simulink model "open_loop_state_estimation"  (R2018b)
settings: Solver=ode2  StartTime=0.0  StopTime=100  FixedStep=0.002  RelTol=1e-3  EnableMultiTasking=on
model workspace (MAT data in the model file):
  m = 1000
undefined symbols (not defined in the file): activate_VariableFriction, sigbuilder_block, tpa_map_Reference, tS, x0_vehiclepose_stm
libraries: simulink x6
settings Model: DataDictionary=controller_dev.sldd  PauseTimes=9.280  Creator=wischnewski  LastModifiedBy=ga25xiw
settings SolverCC: AutoInsertRateTranBlk=on
settings DataIOCC: SaveFormat=StructureWithTime
settings OptimizationCC: BlockReduction=off  DefaultParameterBehavior=Inlined  EnhancedBackFolding=on  PassReuseOutputArgsAs=Individual arguments  OptimizeBlockOrder=speed  DifferentSizesBufferReuse=on  OptimizationCustomize=off
settings DebuggingCC: ParameterTunabilityLossMsg=error
settings HardwareCC: ProdBitPerPointer=32  ProdBitPerSizeT=32  ProdBitPerPtrDiffT=32  ProdLargestAtomicFloat=None  ProdWordSize=32  ProdLongLongMode=on  ProdHWDeviceType=Generic->32-bit x86 compatible
settings ModelReferenceCC: ModelReferenceMinAlgLoopOccurrences=on
settings SFSimCC: SimUseLocalCustomCode=off  MATLABDynamicMemAlloc=off
settings RTWCC: SystemTargetFile=ert.tlc  TemplateMakefile=ert_default_tmf  GenerateReport=on  RTWUseLocalCustomCode=off  IncludeHyperlinkInReport=on  LaunchReport=on  TargetLang=C++  GenerateTraceInfo=on  GenerateTraceReport=on  GenerateTraceReportSl=on  GenerateTraceReportSf=on  GenerateTraceReportEml=on
settings CodeAppCC: ForceParamTrailComments=on  IgnoreCustomStorageClasses=off  OperatorAnnotations=on  SimulinkDataObjDesc=on  SFDataObjDesc=on  InsertBlockDesc=on
settings ERTTargetCC: TargetLangStandard=C++03 (ISO)  GenerateSampleERTMain=on  MultiInstanceERTCode=on  CodeInterfacePackaging=C++ class  InlinedParameterPlacement=NonHierarchical  RootIOFormat=Structure reference  ERTCustomFileTemplate=example_file_process.tlc

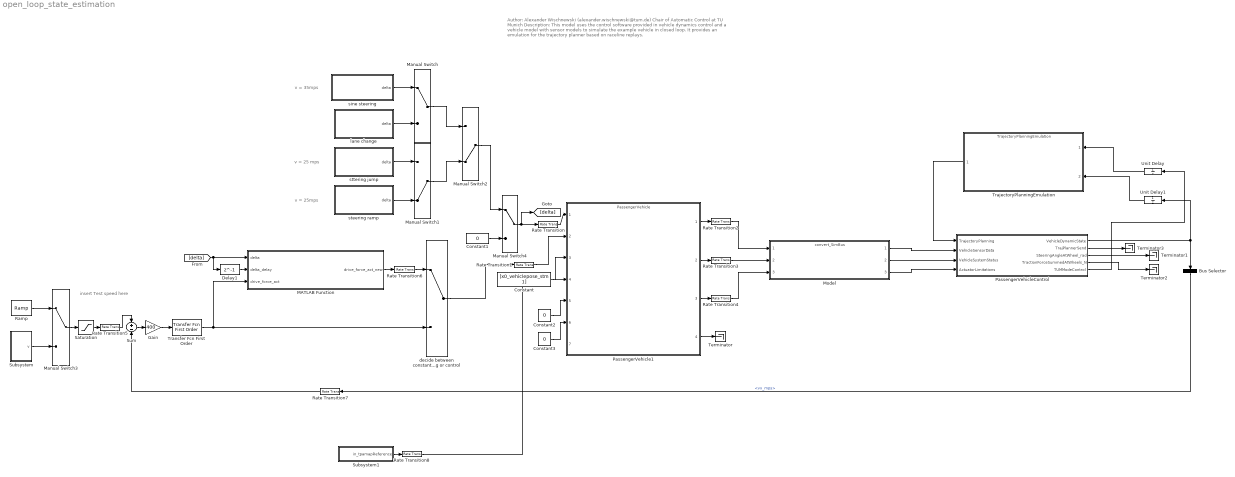
== system open_loop_state_estimation ==
  note: v = 25mps
  note: v = 35mps
  note: v = 25 mps
  note: insert Test speed here
  note: Author: Alexander Wischnewski (alexander.wischnewski@tum.de)
      | Chair of Automatic Control at TU Munich
      |
      | Description: This model uses the control software provided in vehicle dynamics control and a vehicle model
      | with sensor models to simulate the example vehicle in closed loop. It provides an emulation for the trajectory planner based on raceline replays.
  Bus Selector : BusSelector  OutputSignals=vx_mps
  Constant : Constant  Value=[x0_vehiclepose_stm 1]
  Constant1 : Constant  Value=0
  Constant2 : Constant  Value=0
  Constant3 : Constant  Value=0
  Delay1 : Delay  DelayLength=1
  Gain : Gain  Gain=400
  MATLAB Function : MATLAB Function  TreatAsAtomicUnit=on
  Manual Switch : ManualSwitch
  Manual Switch1 : ManualSwitch  CurrentSetting=0
  Manual Switch2 : ManualSwitch  CurrentSetting=0
  Manual Switch3 : ManualSwitch
  Manual Switch4 : ManualSwitch
  Model : ModelReference  ModelNameDialog=convert_SimBus.slx  SimulationMode=Normal  ModelReferenceVersion=1.818
  PassengerVehicle1 : ModelReference  ModelNameDialog=PassengerVehicle  SimulationMode=Normal  ModelReferenceVersion=1.933
  PassengerVehicleControl : Subsystem
  Ramp : simulink/Sources/Ramp  slope=8  start=0  InitialOutput=0.1
  Rate Transition{,1..8} (9 alike) : RateTransition
  Saturation : Saturate  UpperLimit=25  LowerLimit=0
  Subsystem : Subsystem
  Subsystem1 : Subsystem
  Sum : Sum  Inputs=+-
  Terminator{,1..3} (4 alike) : Terminator
  TrajectoryPlanningEmulation : ModelReference  ModelNameDialog=TrajectoryPlanningEmulation.slx  SimulationMode=Normal  ModelReferenceVersion=1.855
  Transfer Fcn First Order : simulink/Discrete/Transfer Fcn First Order  PoleZ=exp(-tS/1)  ICPrevOutput=0.0  DoSatur=off
      settings: SourceProductName=Simulink
  Unit Delay : UnitDelay  SampleTime=-1
  Unit Delay1 : UnitDelay  SampleTime=-1
  "decide between constant torque while steering or control " : ManualSwitch
  lane change : Subsystem
  sine steering : Subsystem
  steering ramp : Subsystem
  sttering jump : Subsystem
  wires:
  TrajectoryPlanningEmulation/1 -> PassengerVehicleControl/1(TrajectoryPlanning)
  PassengerVehicleControl/1(VehicleDynamicState) -> Unit Delay1/1, Bus Selector/1
  Unit Delay/1 -> TrajectoryPlanningEmulation/1
  Unit Delay1/1 -> TrajectoryPlanningEmulation/2
  PassengerVehicle1/3 -> Rate Transition4/1
  PassengerVehicle1/2 -> Rate Transition3/1
  PassengerVehicle1/1 -> Rate Transition2/1
  Constant/1 -> PassengerVehicle1/3
  Rate Transition/1 -> PassengerVehicle1/1
  Rate Transition1/1 -> PassengerVehicle1/2
  PassengerVehicleControl/3(SteeringAngleAtWheel_rad) -> Terminator1/1
  Sum/1 -> Gain/1
  PassengerVehicleControl/4(TractionForceSummedAtWheels_N) -> Terminator2/1
  Bus Selector/1 -> Rate Transition7/1  "<vx_mps>"
  Gain/1 -> Transfer Fcn First Order/1
  Saturation/1 -> Rate Transition5/1
  Rate Transition5/1 -> Sum/1
  sine steering/1(delta) -> Manual Switch/1
  lane change/1(delta) -> Manual Switch/2
  sttering jump/1(delta) -> Manual Switch1/1
  steering ramp/1(delta) -> Manual Switch1/2
  Manual Switch1/1 -> Manual Switch2/2
  Manual Switch/1 -> Manual Switch2/1
  Manual Switch3/1 -> Saturation/1
  Ramp/1 -> Manual Switch3/1
  Manual Switch4/1 -> [delta], Rate Transition/1
  Manual Switch2/1 -> Manual Switch4/1
  Constant1/1 -> Manual Switch4/2
  Subsystem/1("v ") -> Manual Switch3/2
  "decide between constant torque while steering or control "/1 -> Rate Transition1/1
  Transfer Fcn First Order/1 -> "decide between constant torque while steering or control "/2, MATLAB Function/3(drive_force_act)
  [delta] -> MATLAB Function/1(delta), Delay1/1
  Delay1/1 -> MATLAB Function/2(delta_delay)
  MATLAB Function/1(drive_force_act_new) -> Rate Transition6/1
  Rate Transition6/1 -> "decide between constant torque while steering or control "/1
  Rate Transition7/1 -> Sum/2
  PassengerVehicle1/4 -> Terminator/1
  Subsystem1/1(in_tpamapReference) -> Rate Transition8/1
  Rate Transition8/1 -> PassengerVehicle1/4
  Rate Transition2/1 -> Model/1
  Model/1 -> PassengerVehicleControl/2(VehicleSensorData)
  Rate Transition3/1 -> Model/2
  Rate Transition4/1 -> Model/3
  Model/2 -> PassengerVehicleControl/3(VehicleSystemStatus)
  Model/3 -> PassengerVehicleControl/4(ActuatorLimitations)
  Constant2/1 -> PassengerVehicle1/5
  Constant3/1 -> PassengerVehicle1/6
  PassengerVehicleControl/5(TUMModeControl) -> Unit Delay/1
  PassengerVehicleControl/2(TrajPlannerSend) -> Terminator3/1

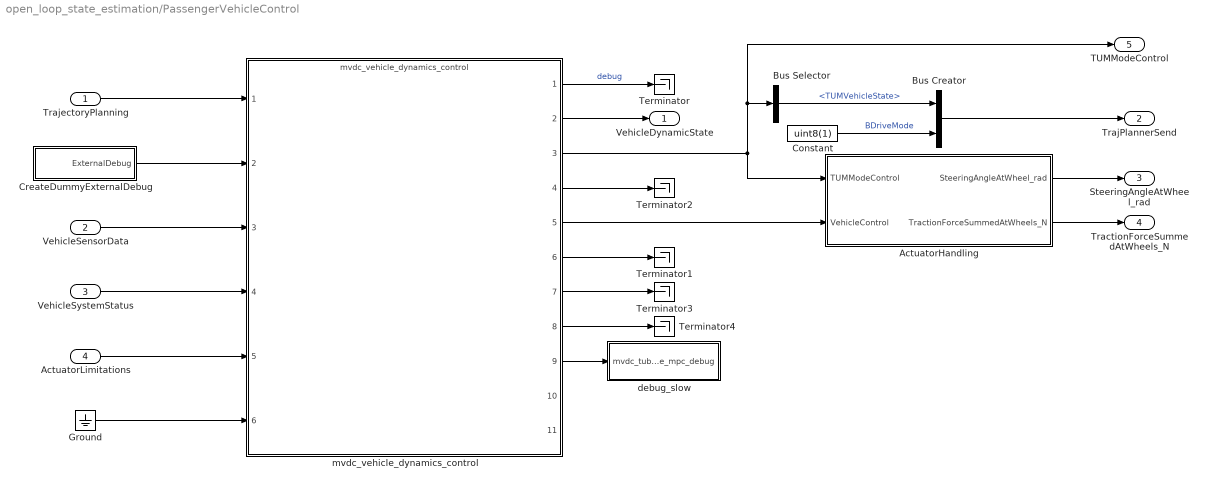
== system open_loop_state_estimation/PassengerVehicleControl ==
  TrajectoryPlanning : Inport
  VehicleSensorData : Inport  Port=2
  VehicleSystemStatus : Inport  Port=3
  ActuatorLimitations : Inport  Port=4
  ActuatorHandling : Subsystem
  Bus Creator : BusCreator  Inputs=2
  Bus Selector : BusSelector  OutputSignals=TUMVehicleState
  Constant : Constant  Value=uint8(1)
  CreateDummyExternalDebug : Subsystem
  Ground : Ground
  Terminator{,1..4} (5 alike) : Terminator
  debug_slow : Subsystem
  mvdc_vehicle_dynamics_control : ModelReference  ModelNameDialog=mvdc_vehicle_dynamics_control  SimulationMode=Normal  ModelReferenceVersion=1.789
  VehicleDynamicState : Outport
  TrajPlannerSend : Outport  Port=2
  SteeringAngleAtWheel_rad : Outport  Port=3
  TractionForceSummedAtWheels_N : Outport  Port=4
  TUMModeControl : Outport  Port=5  OutDataTypeStr=Bus: TUMModeControl
  wires:
  mvdc_vehicle_dynamics_control/1 -> Terminator/1  "debug"
  VehicleSystemStatus/1 -> mvdc_vehicle_dynamics_control/4
  ActuatorLimitations/1 -> mvdc_vehicle_dynamics_control/5
  VehicleSensorData/1 -> mvdc_vehicle_dynamics_control/3
  TrajectoryPlanning/1 -> mvdc_vehicle_dynamics_control/1
  mvdc_vehicle_dynamics_control/5 -> ActuatorHandling/2(VehicleControl)
  mvdc_vehicle_dynamics_control/6 -> Terminator1/1
  ActuatorHandling/2(TractionForceSummedAtWheels_N) -> TractionForceSummedAtWheels_N/1
  ActuatorHandling/1(SteeringAngleAtWheel_rad) -> SteeringAngleAtWheel_rad/1
  mvdc_vehicle_dynamics_control/7 -> Terminator3/1
  mvdc_vehicle_dynamics_control/8 -> Terminator4/1
  Bus Selector/1 -> Bus Creator/1  "<TUMVehicleState>"
  Constant/1 -> Bus Creator/2  "BDriveMode"
  Bus Creator/1 -> TrajPlannerSend/1
  mvdc_vehicle_dynamics_control/2 -> VehicleDynamicState/1
  mvdc_vehicle_dynamics_control/9 -> debug_slow/1(mvdc_tube_mpc_debug)
  mvdc_vehicle_dynamics_control/3 -> ActuatorHandling/1(TUMModeControl), TUMModeControl/1, Bus Selector/1
  mvdc_vehicle_dynamics_control/4 -> Terminator2/1
  CreateDummyExternalDebug/1(ExternalDebug) -> mvdc_vehicle_dynamics_control/2
  Ground/1 -> mvdc_vehicle_dynamics_control/6

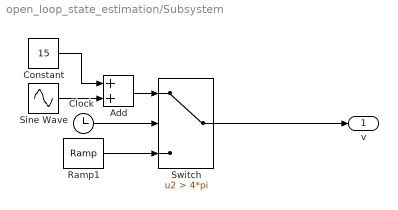
== system open_loop_state_estimation/Subsystem ==
  Add : Sum
  Clock : Clock
  Constant : Constant  Value=15
  Ramp1 : simulink/Sources/Ramp  slope=8  start=0  InitialOutput=0.1
  Sine Wave : Sin  Amplitude=25  SampleTime=0
  Switch : Switch  Criteria=u2 > Threshold  Threshold=4*pi
  "v " : Outport
  wires:
  Clock/1 -> Switch/2
  Switch/1 -> "v "/1
  Ramp1/1 -> Switch/3
  Add/1 -> Switch/1
  Sine Wave/1 -> Add/2
  Constant/1 -> Add/1

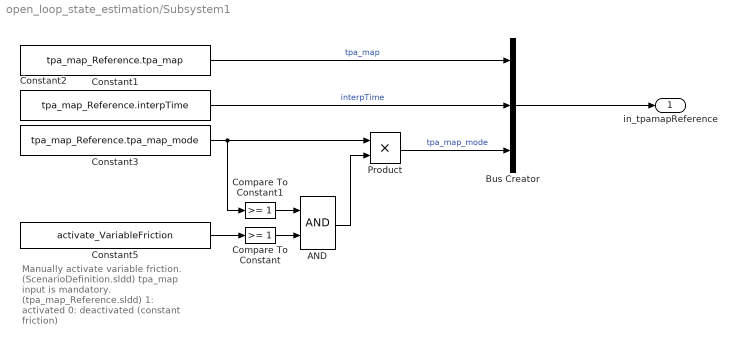
== system open_loop_state_estimation/Subsystem1 ==
  note: Manually activate variable friction.
      | (ScenarioDefinition.sldd)      tpa_map input is mandatory. (tpa_map_Reference.sldd)
      |
      | 1: activated
      | 0: deactivated (constant friction)
  AND : Logic  AllPortsSameDT=off  OutDataTypeStr=boolean
  Bus Creator : BusCreator  Inputs=3  OutDataTypeStr=Bus: tpamapReference
  Compare To Constant : simulink/Logic and Bit Operations/Compare To Constant  relop=>=  const=1  OutDataTypeStr=boolean
  Compare To Constant1 : simulink/Logic and Bit Operations/Compare To Constant  relop=>=  const=1  OutDataTypeStr=boolean
  Constant1 : Constant  Value=tpa_map_Reference.tpa_map
  Constant2 : Constant  Value=tpa_map_Reference.interpTime
  Constant3 : Constant  Value=tpa_map_Reference.tpa_map_mode  OutDataTypeStr=double
  Constant5 : Constant  Value=activate_VariableFriction  OutDataTypeStr=double
  Product : Product  OutDataTypeStr=double
  in_tpamapReference : Outport  OutDataTypeStr=Bus: tpamapReference
  wires:
  Bus Creator/1 -> in_tpamapReference/1
  Constant1/1 -> Bus Creator/1  "tpa_map"
  Constant2/1 -> Bus Creator/2  "interpTime"
  Constant5/1 -> Compare To Constant/1
  Compare To Constant/1 -> AND/2
  Constant3/1 -> Product/1, Compare To Constant1/1
  AND/1 -> Product/2
  Compare To Constant1/1 -> AND/1
  Product/1 -> Bus Creator/3  "tpa_map_mode"

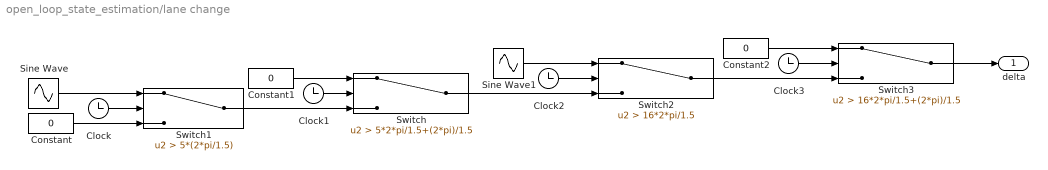
== system open_loop_state_estimation/lane change ==
  Clock{,1..3} (4 alike) : Clock
      settings: Decimation=2
  Constant : Constant  Value=0
  Constant1 : Constant  Value=0
  Constant2 : Constant  Value=0
  Sine Wave : Sin  Amplitude=0.3  Frequency=1.5  SampleTime=0
  Sine Wave1 : Sin  Amplitude=0.3  Frequency=1.5  SampleTime=0
  Switch : Switch  Criteria=u2 > Threshold  Threshold=5*2*pi/1.5+(2*pi)/1.5
  Switch1 : Switch  Criteria=u2 > Threshold  Threshold=5*(2*pi/1.5)
  Switch2 : Switch  Criteria=u2 > Threshold  Threshold=16*2*pi/1.5
  Switch3 : Switch  Criteria=u2 > Threshold  Threshold=16*2*pi/1.5+(2*pi)/1.5
  delta : Outport
  wires:
  Switch1/1 -> Switch/3
  Sine Wave/1 -> Switch1/1
  Clock/1 -> Switch1/2
  Clock1/1 -> Switch/2
  Constant/1 -> Switch1/3
  Constant1/1 -> Switch/1
  Switch/1 -> Switch2/3
  Clock2/1 -> Switch2/2
  Sine Wave1/1 -> Switch2/1
  Switch2/1 -> Switch3/3
  Clock3/1 -> Switch3/2
  Constant2/1 -> Switch3/1
  Switch3/1 -> delta/1

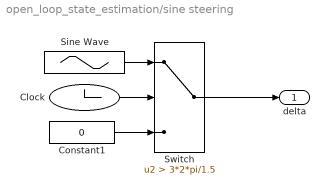
== system open_loop_state_estimation/sine steering ==
  Clock : Clock
      settings: Decimation=2
  Constant1 : Constant  Value=0
  Sine Wave : Sin  Amplitude=0.3  Frequency=1.5  SampleTime=0
  Switch : Switch  Criteria=u2 > Threshold  Threshold=3*2*pi/1.5
  delta : Outport
  wires:
  Constant1/1 -> Switch/3
  Clock/1 -> Switch/2
  Sine Wave/1 -> Switch/1
  Switch/1 -> delta/1

== system open_loop_state_estimation/steering ramp ==
  Signal Builder : Subsystem  Tag=STV Subsys  LoadFcn=sigbuilder_block('load');  StartFcn=sigbuilder_block('start');  StopFcn=sigbuilder_block('stop');  ClipboardFcn=sigbuilder_block('clipboard');  mask(Sigbuilder block){tuvar=[0:10]}
      mask help: Simulink:masks:SigbuilderBlock_MD
      mask init:
      | if ~strcmp(get_param(bdroot(gcbh),'SimulationStatus'),'stopped') tuvar = sigbuilder_block('maskInit'); end
      settings: CopyFcn=sigbuilder_block('copy');  DeleteFcn=sigbuilder_block('delete');  ModelCloseFcn=sigbuilder_block('modelClose');  PreSaveFcn=sigbuilder_block('preSave');  PauseFcn=sigbuilder_block('pause');  ContinueFcn=sigbuilder_block('continue');  NameChangeFcn=sigbuilder_block('namechange');  OpenFcn=sigbuilder_block('open',[6 22.5 1428 689.25 ]);  CloseFcn=sigbuilder_block('close');
      mask Display: plot(0, 0, 100, 100,[2, 2, 32, 32, 2], [68, 8, 8, 68, 68],[32, 2], [38, 38], [32, 19, 2],[53, 60, 44], [32, 17, 17, 2],[16, 16, 31, 31]);txt = getActiveGroup(gcbh);text(2, 100, txt,'verticalAlignment', 'top');
  delta : Outport
  wires:
  Signal Builder/1(Signal 1) -> delta/1

== system open_loop_state_estimation/sttering jump ==
  Signal Builder : Subsystem  Tag=STV Subsys  LoadFcn=sigbuilder_block('load');  StartFcn=sigbuilder_block('start');  StopFcn=sigbuilder_block('stop');  ClipboardFcn=sigbuilder_block('clipboard');  mask(Sigbuilder block){tuvar=[0:10]}
      mask help: Simulink:masks:SigbuilderBlock_MD
      mask init:
      | if ~strcmp(get_param(bdroot(gcbh),'SimulationStatus'),'stopped') tuvar = sigbuilder_block('maskInit'); end
      settings: CopyFcn=sigbuilder_block('copy');  DeleteFcn=sigbuilder_block('delete');  ModelCloseFcn=sigbuilder_block('modelClose');  PreSaveFcn=sigbuilder_block('preSave');  PauseFcn=sigbuilder_block('pause');  ContinueFcn=sigbuilder_block('continue');  NameChangeFcn=sigbuilder_block('namechange');  OpenFcn=sigbuilder_block('open',[6 22.5 1428 689.25 ]);  CloseFcn=sigbuilder_block('close');
      mask Display: plot(0, 0, 100, 100,[2, 2, 32, 32, 2], [68, 8, 8, 68, 68],[32, 2], [38, 38], [32, 19, 2],[53, 60, 44], [32, 17, 17, 2],[16, 16, 31, 31]);txt = getActiveGroup(gcbh);text(2, 100, txt,'verticalAlignment', 'top');
  delta : Outport
  wires:
  Signal Builder/1(Signal 1) -> delta/1

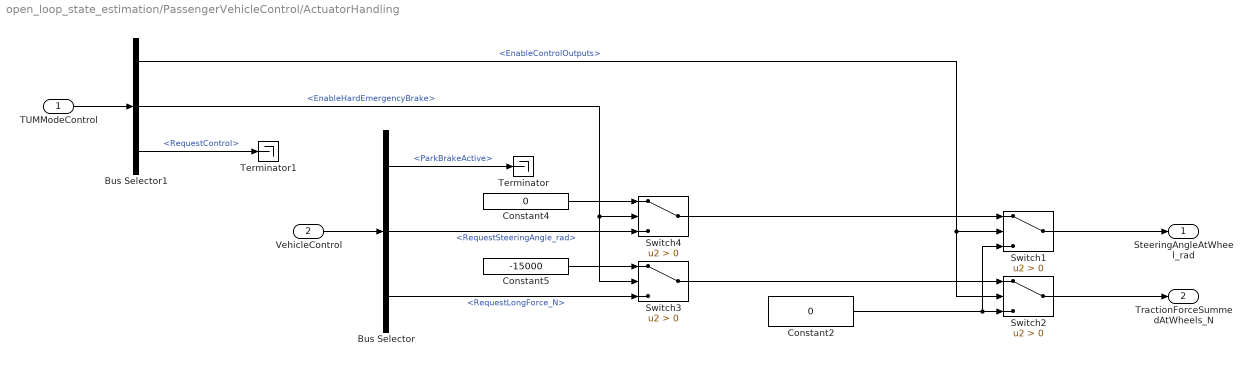
== system open_loop_state_estimation/PassengerVehicleControl/ActuatorHandling ==
  TUMModeControl : Inport  OutDataTypeStr=Bus: TUMModeControl
  VehicleControl : Inport  Port=2  OutDataTypeStr=Bus: VehicleControl
  Bus Selector : BusSelector  OutputSignals=ParkBrakeActive,RequestSteeringAngle_rad,RequestLongForce_N
  Bus Selector1 : BusSelector  OutputSignals=EnableControlOutputs,EnableHardEmergencyBrake,RequestControl
  Constant2 : Constant  Value=0
  Constant4 : Constant  Value=0
  Constant5 : Constant  Value=-15000
  Switch{1..4} (4 alike) : Switch  Criteria=u2 > Threshold
  Terminator : Terminator
  Terminator1 : Terminator
  SteeringAngleAtWheel_rad : Outport
  TractionForceSummedAtWheels_N : Outport  Port=2
  wires:
  Bus Selector1/1 -> Switch2/2, Switch1/2  "<EnableControlOutputs>"
  TUMModeControl/1 -> Bus Selector1/1
  Bus Selector/3 -> Switch3/3  "<RequestLongForce_N>"
  Constant2/1 -> Switch1/3, Switch2/3
  VehicleControl/1 -> Bus Selector/1
  Bus Selector/2 -> Switch4/3  "<RequestSteeringAngle_rad>"
  Constant4/1 -> Switch4/1
  Constant5/1 -> Switch3/1
  Bus Selector1/2 -> Switch3/2, Switch4/2  "<EnableHardEmergencyBrake>"
  Bus Selector/1 -> Terminator/1  "<ParkBrakeActive>"
  Bus Selector1/3 -> Terminator1/1  "<RequestControl>"
  Switch4/1 -> Switch1/1
  Switch3/1 -> Switch2/1
  Switch1/1 -> SteeringAngleAtWheel_rad/1
  Switch2/1 -> TractionForceSummedAtWheels_N/1

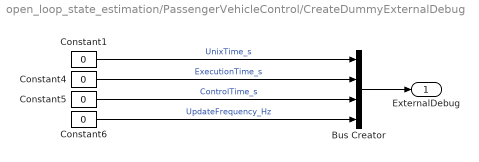
== system open_loop_state_estimation/PassengerVehicleControl/CreateDummyExternalDebug ==
  Bus Creator : BusCreator  Inputs=4
  Constant{1,4..6} (4 alike) : Constant  Value=0
  ExternalDebug : Outport  OutDataTypeStr=Bus: ExternalDebug
  wires:
  Constant1/1 -> Bus Creator/1  "UnixTime_s"
  Constant4/1 -> Bus Creator/2  "ExecutionTime_s"
  Constant6/1 -> Bus Creator/4  "UpdateFrequency_Hz"
  Constant5/1 -> Bus Creator/3  "ControlTime_s"
  Bus Creator/1 -> ExternalDebug/1

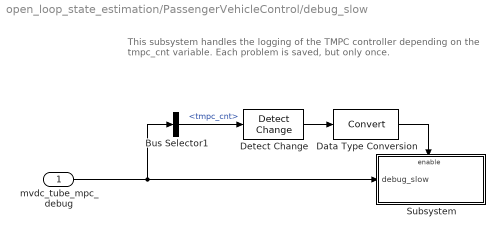
== system open_loop_state_estimation/PassengerVehicleControl/debug_slow ==
  note: This subsystem handles the logging of the TMPC controller
      | depending on the tmpc_cnt variable. Each problem is saved, but only once.
  mvdc_tube_mpc_debug : Inport
  Bus Selector1 : BusSelector  OutputSignals=tmpc_cnt
  Data Type Conversion : DataTypeConversion
  Detect Change : simulink/Logic and Bit Operations/Detect Change  vinit=0  OutDataTypeStr=boolean
  Subsystem : Subsystem
  wires:
  Detect Change/1 -> Data Type Conversion/1
  Data Type Conversion/1 -> Subsystem/Enable
  mvdc_tube_mpc_debug/1 -> Bus Selector1/1, Subsystem/1(debug_slow)
  Bus Selector1/1 -> Detect Change/1  "<tmpc_cnt>"

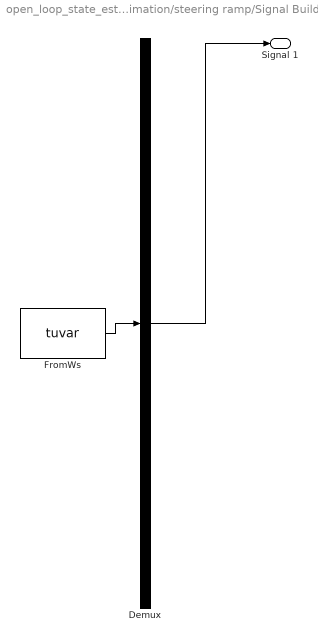
== system open_loop_state_estimation/steering ramp/Signal Builder ==
  Demux : Demux  Tag=STV Demux  Outputs=1
  FromWs : FromWorkspace  Tag=STV FromWs  VariableName=tuvar  SampleTime=0
      SigBuilderData=|
      | common.afterFinalStr = 'Extrapolate'
      | common.sampleTime = 0
      | dataSet.timeRange = [0 100]
      | dataSet.name = 'Group 1'
      | sbobj.Groups.Name = 'Group 1'
      | sbobj.Groups.Signals.Name = 'Signal 1'
      | sbobj.Groups.Signals.XData = [0 20 30 40 50 60 70 100]
      | sbobj.Groups.Signals.YData = [0 0 -0.3 0 0 0.3 -0.000505 0]
      | sbobj.Groups.TimeRange = [0 100]
  Signal 1 : Outport  Tag=STV Outport
  wires:
  FromWs/1 -> Demux/1
  Demux/1 -> Signal 1/1

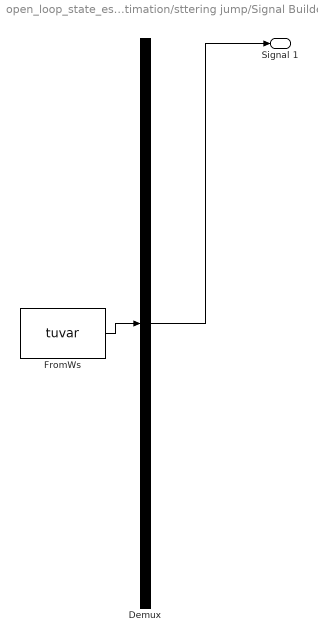
== system open_loop_state_estimation/sttering jump/Signal Builder ==
  Demux : Demux  Tag=STV Demux  Outputs=1
  FromWs : FromWorkspace  Tag=STV FromWs  VariableName=tuvar  SampleTime=0
      SigBuilderData=|
      | common.afterFinalStr = 'Extrapolate'
      | common.sampleTime = 0
      | dataSet.timeRange = [0 100]
      | dataSet.name = 'Group 1'
      | sbobj.Groups.Name = 'Group 1'
      | sbobj.Groups.Signals.Name = 'Signal 1'
      | sbobj.Groups.Signals.XData = [0 15 15.5 40 40 60 60.6 85 85 100]
      | sbobj.Groups.Signals.YData = [0 0 0.3 0.302 0 0 -0.3 -0.3 0 0]
      | sbobj.Groups.TimeRange = [0 100]
  Signal 1 : Outport  Tag=STV Outport
  wires:
  Demux/1 -> Signal 1/1
  FromWs/1 -> Demux/1

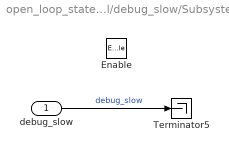
== system open_loop_state_estimation/PassengerVehicleControl/debug_slow/Subsystem ==
  debug_slow : Inport
  Enable : EnablePort
  Terminator5 : Terminator
  wires:
  debug_slow/1 -> Terminator5/1  "debug_slow"

== matlab function open_loop_state_estimation/MATLAB Function ==
  settings: updateMethod=DISCRETE
  data: delta input; delta_delay input; drive_force_act input; drive_force_act_new output
function drive_force_act_new = get_constant_drive_force(delta, delta_delay, drive_force_act)

persistent temp

if isempty(temp)
    temp = zeros(2,1);
end


 if delta_delay == 0 && abs(delta) > 0
        temp(2) = drive_force_act;
 else
        temp(1) = 0;
 end
 
 if abs(delta) > 0
     drive_force_act_new = max(temp);
 else
     drive_force_act_new = drive_force_act;
 end
